simulink model "untitled"  (R2021b)
settings: Solver=VariableStepAuto  StartTime=0.0  StopTime=10.0  RelTol=1e-3
undefined symbols (not defined in the file or in its folder): Earth, WGS84
libraries: aerolibtransform2 x1
settings Model: Creator=Shiyu Cheng  LastModifiedBy=Shiyu Cheng

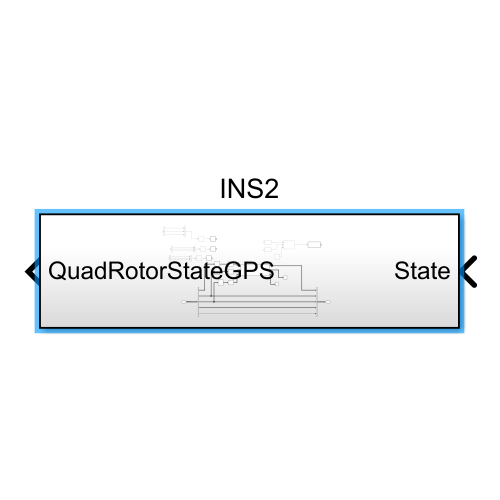
[thumbnail: Simulink's stored preview of the top-level diagram]
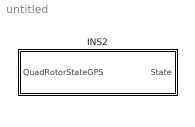
== system untitled ==
  INS2 : Subsystem

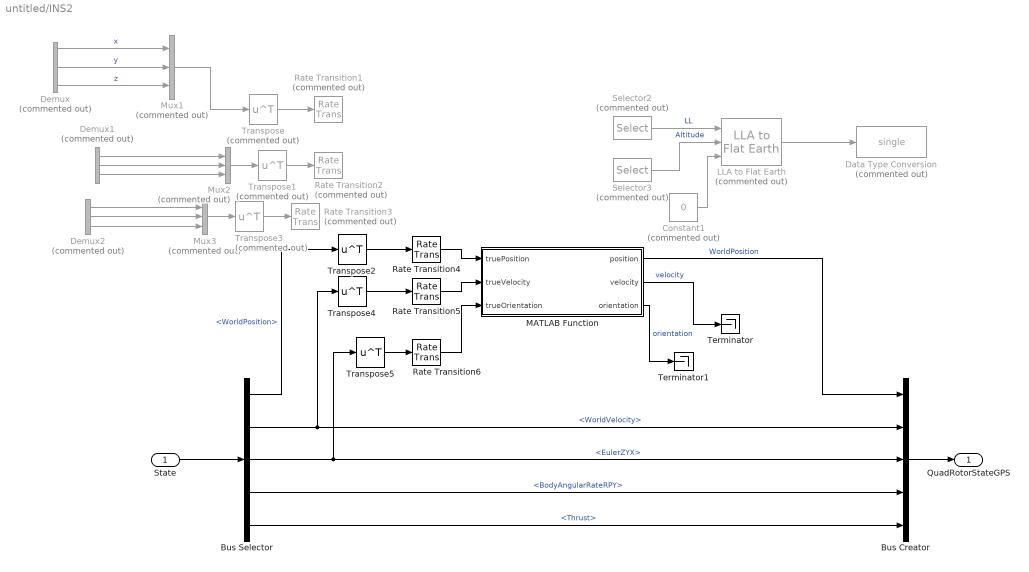
== system untitled/INS2 ==
  State : Inport
  Bus Creator : BusCreator  Inputs=5
  Bus Selector : BusSelector  OutputSignals=WorldPosition,WorldVelocity,EulerZYX,BodyAngularRateRPY,Thrust
  Constant1 : Constant  Commented=on  Value=0
  Data Type Conversion : DataTypeConversion  Commented=on  OutDataTypeStr=single
  Demux : Demux  Commented=on  Outputs=3
  Demux1 : Demux  Commented=on  Outputs=3
  Demux2 : Demux  Commented=on  Outputs=3
  LLA to Flat Earth : aerolibtransform2/LLA to Flat Earth  Commented=on  units=Metric (MKS)  ptype=Earth (WGS84)  F=1/298.257223563  R=6378137  refPosPort=off  LL0=[41.8856528 -87.6556726]  psi=0
      settings: SourceProductBaseCode=AE
  MATLAB Function : MATLAB Function  TreatAsAtomicUnit=on
  Mux1 : Mux  Commented=on  Inputs=3
  Mux2 : Mux  Commented=on  Inputs=3
  Mux3 : Mux  Commented=on  Inputs=3
  Rate Transition1 : RateTransition  Commented=on  OutPortSampleTime=UAVSampleTime
  Rate Transition2 : RateTransition  Commented=on  OutPortSampleTime=UAVSampleTime
  Rate Transition3 : RateTransition  Commented=on  OutPortSampleTime=UAVSampleTime
  Rate Transition4 : RateTransition  OutPortSampleTime=UAVSampleTime
  Rate Transition5 : RateTransition  OutPortSampleTime=UAVSampleTime
  Rate Transition6 : RateTransition  OutPortSampleTime=UAVSampleTime
  Selector2 : Selector  Commented=on  InputPortWidth=3  IndexOptions=Index vector (dialog)  Indices=[1 2]  OutputSizes=1
  Selector3 : Selector  Commented=on  InputPortWidth=3  IndexOptions=Index vector (dialog)  Indices=[3]  OutputSizes=1
  Terminator : Terminator
  Terminator1 : Terminator
  Transpose : Math  Commented=on  Operator=transpose  SaturateOnIntegerOverflow=on
  Transpose1 : Math  Commented=on  Operator=transpose  SaturateOnIntegerOverflow=on
  Transpose2 : Math  Operator=transpose  SaturateOnIntegerOverflow=on
  Transpose3 : Math  Commented=on  Operator=transpose  SaturateOnIntegerOverflow=on
  Transpose4 : Math  Operator=transpose  SaturateOnIntegerOverflow=on
  Transpose5 : Math  Operator=transpose  SaturateOnIntegerOverflow=on
  QuadRotorStateGPS : Outport
  wires:
  State/1 -> Bus Selector/1
  Bus Creator/1 -> QuadRotorStateGPS/1
  Bus Selector/2 -> Transpose4/1, Bus Creator/2  "<WorldVelocity>"
  Bus Selector/3 -> Bus Creator/3, Transpose5/1  "<EulerZYX>"
  Bus Selector/4 -> Bus Creator/4  "<BodyAngularRateRPY>"
  Bus Selector/5 -> Bus Creator/5  "<Thrust>"
  Demux/1 -> Mux1/1  "x"
  Transpose/1 -> Rate Transition1/1
  Selector3/1 -> LLA to Flat Earth/2  "Altitude"
  Selector2/1 -> LLA to Flat Earth/1  "LL"
  MATLAB Function/3(orientation) -> Terminator1/1  "orientation"
  Mux2/1 -> Transpose1/1
  Mux1/1 -> Transpose/1
  Constant1/1 -> LLA to Flat Earth/3
  LLA to Flat Earth/1 -> Data Type Conversion/1
  Transpose1/1 -> Rate Transition2/1
  MATLAB Function/2(velocity) -> Terminator/1  "velocity"
  Mux3/1 -> Transpose3/1
  Transpose3/1 -> Rate Transition3/1
  Demux2/3 -> Mux3/3
  Demux/2 -> Mux1/2  "y"
  Demux/3 -> Mux1/3  "z"
  Demux1/1 -> Mux2/1
  Demux1/2 -> Mux2/2
  Demux1/3 -> Mux2/3
  Demux2/1 -> Mux3/1
  Demux2/2 -> Mux3/2
  Bus Selector/1 -> Transpose2/1  "<WorldPosition>"
  Transpose2/1 -> Rate Transition4/1
  Rate Transition4/1 -> MATLAB Function/1(truePosition)
  Transpose4/1 -> Rate Transition5/1
  Rate Transition5/1 -> MATLAB Function/2(trueVelocity)
  Transpose5/1 -> Rate Transition6/1
  Rate Transition6/1 -> MATLAB Function/3(trueOrientation)
  MATLAB Function/1(position) -> Bus Creator/1  "WorldPosition"

== matlab function untitled/INS2/MATLAB Function ==
  data: truePosition input; position output; trueVelocity input; velocity output; orientation output; trueOrientation input
function [position, velocity, orientation] = simINS(truePosition,trueVelocity,trueOrientation)
gTruth = struct('Position',truePosition,'Velocity',trueVelocity,'Orientation',trueOrientation);
% INS = insSensor("PositionAccuracy",[0.1 0.1 0.1],'RollAccuracy',0,...
%     'PitchAccuracy',0,'VelocityAccuracy',0,'YawAccuracy',0);
INS = insSensor('RollAccuracy',0,'PitchAccuracy',0,'YawAccuracy',0,'PositionAccuracy',[0 0 0],...
    'VelocityAccuracy',0,'AccelerationAccuracy',0);
insMeas = INS(gTruth);
position = insMeas.Position;
x =  position(1);
y = -position(2);
if y <= 100
    x = x - 20;
end
position(1) = x;
velocity = insMeas.Velocity;
orientation = insMeas.Orientation;
end
